simulink model "KalmanWienerFilterExample"  (R2019b)
settings: Solver=VariableStepAuto  StartTime=0.0  StopTime=10.0  RelTol=1e-3
undefined symbols (not defined in the file or in its folder): A_cont, B_cont, C_cont, D_cont, DiscIntNeverNeededParam, Discrete, L, q, r, Time
libraries: simulink x2, ctrlSharedLib x1
settings Model: Creator=Sankalp Bhan  LastModifiedBy=cwhipp

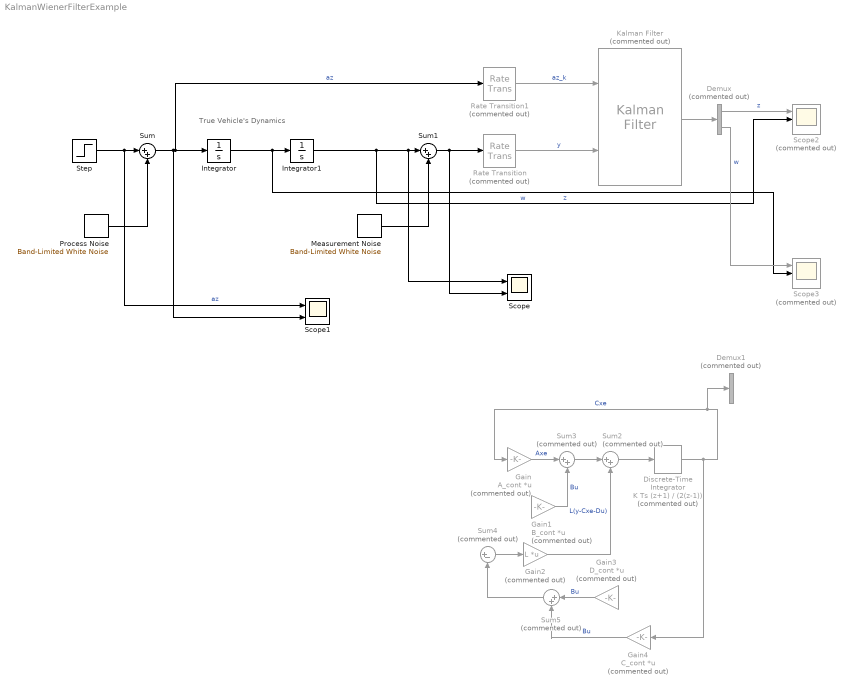
== system KalmanWienerFilterExample ==
  note: True Vehicle's Dynamics
  Demux : Demux  Commented=on  Outputs=2
  Demux1 : Demux  Commented=on  Outputs=2
  Discrete-Time Integrator : DiscreteIntegrator  Commented=on  IntegratorMethod=Integration: Trapezoidal  SampleTime=-1  ICPrevOutput=DiscIntNeverNeededParam  ICPrevScaledInput=DiscIntNeverNeededParam
  Gain : Gain  Commented=on  Gain=A_cont  Multiplication=Matrix(K*u)
  Gain1 : Gain  Commented=on  Gain=B_cont  Multiplication=Matrix(K*u)
  Gain2 : Gain  Commented=on  Gain=L  Multiplication=Matrix(K*u)
  Gain3 : Gain  Commented=on  Gain=D_cont  Multiplication=Matrix(K*u)
  Gain4 : Gain  Commented=on  Gain=C_cont  Multiplication=Matrix(K*u)
  Integrator : Integrator
  Integrator1 : Integrator
  Kalman Filter : ctrlSharedLib/Kalman Filter  Commented=on  TimeDomain=Discrete-Time  UseCurrentEstimator=on  ModelSource=Individual A, B, C, D matrices  ModelSourceVariable=ss(0.95,1,1,0,1)  A=[1 0.005 ; 0 1]  B="[0.005^2/2 ;  0.005]"  C=[1 0]  D=0  NumberOfStates=1  NumberOfInputs=1  NumberOfOutputs=1  InitialEstimateSource=Dialog  X0=[0;0 ]  P0=10  UseK=off  UseGH=off  NumberOfProcessNoiseInputs=1  G=1  TimeInvariantG=on  H=0  TimeInvariantH=on  Q=[0 0 ; 0 1]*q;  TimeInvariantQ=on  R=10*r;  TimeInvariantR=on  N=0  TimeInvariantN=on  AddInputPort=on  AddEnablePort=off  OutputEstimatedY=off  OutputP=off  Ts=-1
      settings: SourceProductBaseCode=CT
  Measurement Noise : simulink/Sources/Band-Limited White Noise  Cov=[0.1]  Ts=0.005  seed=[23341]
  Process Noise : simulink/Sources/Band-Limited White Noise  Cov=[0.1]  Ts=0.005  seed=[23342]
  Rate Transition : RateTransition  Commented=on  OutPortSampleTime=0.005
  Rate Transition1 : RateTransition  Commented=on  OutPortSampleTime=0.005
  Scope : Scope  NumInputPorts=2
  Scope1 : Scope  NumInputPorts=2
  Scope2 : Scope  Commented=on  NumInputPorts=3
  Scope3 : Scope  Commented=on  NumInputPorts=3
  Step : Step  SampleTime=0
  Sum : Sum  Inputs=|++
  Sum1 : Sum  Inputs=|++
  Sum2 : Sum  Commented=on  Inputs=|++
  Sum3 : Sum  Commented=on  Inputs=|++
  Sum4 : Sum  Commented=on  Inputs=|+-
  Sum5 : Sum  Commented=on  Inputs=|++
  wires:
  Integrator/1 -> Scope3/2, Integrator1/1  "w"
  Rate Transition/1 -> Kalman Filter/2  "y"
  Step/1 -> Scope1/1, Sum/1  "az"
  Process Noise/1 -> Sum/2
  Sum1/1 -> Scope/2, Rate Transition/1
  Measurement Noise/1 -> Sum1/2
  Integrator1/1 -> Scope2/2, Scope/1, Sum1/1  "z"
  Rate Transition1/1 -> Kalman Filter/1  "az_k"
  Kalman Filter/1 -> Demux/1
  Demux/1 -> Scope2/1  "z"
  Demux/2 -> Scope3/1  "w"
  Gain/1 -> Sum3/1  "Axe"
  Sum/1 -> Scope1/2, Rate Transition1/1, Integrator/1  "az"
  Gain1/1 -> Sum3/2  "Bu"
  Discrete-Time Integrator/1 -> Gain4/1, Demux1/1, Gain/1  "Cxe"
  Sum3/1 -> Sum2/1
  Sum2/1 -> Discrete-Time Integrator/1
  Gain2/1 -> Sum2/2  "L(y-Cxe-Du)"
  Sum4/1 -> Gain2/1
  Sum5/1 -> Sum4/2
  Gain3/1 -> Sum5/1  "Bu"
  Gain4/1 -> Sum5/2  "Bu"
